simulink model "satcorr_108"  (Simulink 6.2)
settings: Solver=ode45  StartTime=0.0  StopTime=5000  RelTol=1e-3
undefined symbols (not defined in the file): cmult_4bit_br, cmult_4bit_em, cmult_4bit_sl
libraries: xbsIndex_r3 x473, casper_library x42, xps_library x31, ddc_library x4, fft_library x2, pfb_library x2, simulink x1
(part 1 of 5)
settings Model: LastModifiedBy=siemion
settings DebuggingCC: SolverPrmCheckMsg=warning

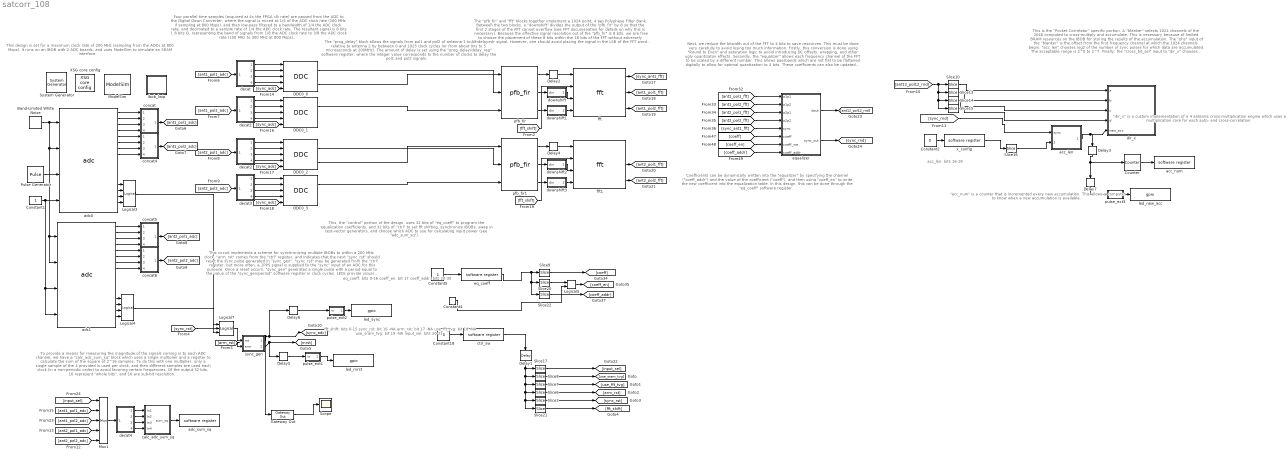
== system satcorr_108 ==
  note: fft_shift: bits 0-15
      | sync_rst: bit 16 -NA
      | arm_rst: bit 17 -NA
      | use_fft_tvg: bit 18 -NA
      | use_sram_tvg: bit 19 -NA
      | input_sel: bits 20-21
  note: acc_len: bits 16-18
  note: eq_coeff: bits 0-16
      | coeff_en: bit 17
      | coeff_addr: bits 20-30
  note: This design is set for a maximum
      | clock rate of 200 MHz (sampling
      | from the ADCs at 800 Mxps).  It
      | runs on an IBOB with 2 ADC boards,
      | and uses ModelSim to simulate an
      | SRAM interface.
  note: This circuit implements a scheme for synchronizing
      | multiple IBOBs to within a 200 MHz clock.  "arm_rst"
      | comes from the "ctrl" register, and indicates that the
      | next "sync_rst" should reset the sync pulse generated
      | in "sync_gen".  "sync_rst" may be generated from
      | the "ctrl" register, but more often, a 1PPS signal is
      | supplied to the "sync" input of an ADC for this
      | purpose.  Once a reset occurs, "sync_gen" generates
      | a single pulse with a period equal to the value
      | of the "sync_gen/period" software register in clock
      | cycles. LEDs provide visual confirmation that an arm and
      | reset occur.
  note: Four parallel time samples (acquired at 4x the
      | FPGA clk rate) are passed from the ADC to the
      | Digital Down Converter, where the signal is mixed
      | at 1/4 of the ADC clock rate (200 MHz if sampling
      | at 800 Msps), and then low-pass filtered to a
      | bandwidth of 1/4 the ADC clock rate, and decimated
      | to a sample rate of 1/4 the ADC clock rate.  The
      | resultant signal is 8 bits I, 8 bits Q, representing the
      | band of signals from 1/8 the ADC clock rate to
      | 3/8 the ADC clock rate (100 MHz to 300 MHz at
      | 800 Msps).
  note: The "pfb_fir" and "fft" blocks together implement a 1024 point,
      | 4 tap Polyphase Filter Bank.  Between the two blocks, a "downshift"
      | divides the output of the "pfb_fir" by 8 so that the first 2 stages of
      | the FFT cannot overflow (see FFT documenation for details on why
      | this is necessary).  Because the effective signal resolution out of
      | the "pfb_fir" is 8 bits, we are free to choose the placement of
      | these 8 bits within the 18 bits of the FFT without adversely affecting
      | our signal.  However, one should avoid placing the signal in the LSB
      | of the FFT word because of rounding effects.  Thus, we downshift
      | only 3 bits.
  note: Next, we reduce the bitwidth out of the FFT to 4 bits to save resources.
      | This must be done very carefully to avoid losing too much information.
      | Firstly, this conversion is done using "Round to Even" and saturation
      | logic to avoid introducing DC offsets, wrapping, and other ugly quantizaton
      | effects.  Secondly, the "equalizer" allows each frequency channel of the
      | FFT to be scaled by a different number.  This allows passbands which are
      | not flat to be flattened digitally to allow for optimal quantization to 4 bits.
      | These coefficients can also be updated dynamically for gain control.
  note: Coefficients can be dynamically written into the "equalizer" by
      | specifying the channel ("coeff_addr") and the value of the
      | coefficient ("coeff"), and then using "coeff_en" to write the
      | new coefficient into the equalization table.  In this design,
      | this can be done through the "eq_coeff" software
      | register.
  note: To provide a means for measuring the magnitude of the signals
      | coming in to each ADC channel, we have a "calc_adc_sum_sq"
      | block which uses a single multiplier and a regsiter to calculate
      | the sum of the square of 2^16 samples.  To do this with one
      | multiplier, only a single sample of the 4 provided is used
      | per clock, and then different samples are used each clock (in
      | a non-periodic order) to avoid favoring certain frequencies.
      | Of the output 32 bits, 16 represent "whole bits", and 16
      | are sub-bit resolution.
  note: This is the "Pocket Correlator" specific portion.  A "blanker" selects
      | 1024 channels of the 2048 computed to cross-multiply and accumulate.
      | This is necessary because of limited BRAM resources on the IBOB
      | for storing the results of the accumulation.  The "phs" input of the "blanker"
      | is the offset from the first frequency channel at which the 1024 channels begin.
      | "acc_len" chooses log2 of the  number of sync pulses for which data are
      | accumulated.  The acceptable range is 2^0 to 2^7.  Finally, the "cross_bit_sel"
      | input to "dir_x" chooses which 16 bits of the 32 accumulated bits are written
      | to the BRAM output buffer.  Only 16 bits real, 16 imag are passed along
      | to reduce download time over the serial cable to a computer.  Which 16 of
      | the 32 computed bits are passed along needs to be selectable because
      | highly correlated signals will accumulate to much larger values than
      | uncorrelated signals.  Values of "cross_bit_sel" can be 0,1,2 or 3
      | corresponding to offsets of 4, 8, 12, and 16 bits from the LSB.
  note: "dir_x" is a custom implementation
      | of a 4 antenna cross-multiplication
      | engine which uses a multiplication
      | core for each auto- and cross-correlation.
  note: "acc_num" is a counter that is
      | incremented every new accumulation.
      | This allows a computer to know when
      | a new accumulation is available.
  note: This, the "control" portion of the design, uses
      | 32 bits of "eq_coeff" to program the equalization
      | coefficients, and 32 bits of "ctrl" to set fft shifting,
      | synchronize IBOBs, swap in test-vector generators,
      | and choose which ADC to use for calculating
      | input power (see "adc_sum_sq").
  note: The "prog_delay" block allows the signals from pol1 and pol2 of antenna 1 to be
      | delayed relative to antenna 2 by between 0 and 1023 clock cycles (or from about
      | 0ns to 5 microseconds at 200MHz).  The amount of delay is set using the
      | "prog_delay/delay_reg" software register, where the integer value corresponds to
      | the number of clocks to delay the pol1 and pol2 signals.
  " System Generator" : xbsIndex_r3/ System Generator  Tag=genX  xilinxfamily=Virtex2P  part=xc2vp50  speed=-7  package=ff1152  synthesis_tool=XST  directory=./satcorr_1/sysgen  testbench=off  simulink_period=1  sysclk_period=41.6667  incr_netlist=off  trim_vbits=Everywhere in SubSystem  dbl_ovrd=According to Block Masks  core_generation=According to Block Masks  run_coregen=off  deprecated_control=off  eval_field=0
      settings: AttributesFormatString=System\nGenerator
  Band-Limited White Noise : simulink/Sources/Band-Limited White Noise  Cov=[0.1]  Ts=0.1  seed=[23341]
  Constant1 : Constant
  Constant18 : Constant  Value=0
  Constant2 : Constant  Value=0
  Constant4 : xbsIndex_r3/Constant  const=1  equ=P=C  arith_type=Boolean  n_bits=1  bin_pt=0  opselect=C  inp2=PCIN>>17  opr=+  inp1=P  carry=CIN  iostate=0  explicit_period=on  period=1  dbl_ovrd=off
  Constant5 : Constant
  Counter : xbsIndex_r3/Counter  cnt_type=Free Running  n_bits=32  bin_pt=0  arith_type=Unsigned  start_count=0  cnt_to=Inf  cnt_by_val=1  operation=Up  explicit_period=off  period=1  load_pin=off  rst=off  en=on  dbl_ovrd=off  show_param=off  use_rpm=on  gen_core=off
      settings: xl_area=[0, 0, 0, 0, 0, 0, 0]
  DDC0_{0..3} (4 alike) : ddc_library/DDC  freq_div=4  lo_freq=1  num_inputs=4  lo_bitwidth=8  lpfir_coeff=".9 * [-0.0161   -0.0428   -0.0504   -0.0249    0.0354    0.1170    0.1948    0.2422    0.2422    0.1948    0.1170  0.0354   -0.0249   -0.0504   -0.0428   -0.0161]"  BitWidthOut=8  quantization="Round  (unbiased: Even Values)"  add_latency=2  mult_latency=4
  Delay1 : xbsIndex_r3/Delay  Orientation=down  latency=1  reg_retiming=off  explicit_period=off  period=1  en=off  accept_only_valid=off  init_zero=on  dbl_ovrd=off  show_param=off
      settings: xl_area=[0, 0, 0, 0, 0, 0, 0]
  Delay2 : xbsIndex_r3/Delay  latency=2  reg_retiming=off  explicit_period=off  period=1  en=off  accept_only_valid=off  init_zero=on  dbl_ovrd=off  show_param=off
      settings: xl_area=[0, 0, 0, 0, 0, 0, 0]
  Delay3 : xbsIndex_r3/Delay  Orientation=down  latency=4  reg_retiming=on  explicit_period=off  period=1  en=off  accept_only_valid=off  init_zero=on  dbl_ovrd=off  show_param=on
      settings: xl_area=[0, 0, 0, 0, 0, 0, 0]
  Delay4 : xbsIndex_r3/Delay  latency=2  reg_retiming=off  explicit_period=off  period=1  en=off  accept_only_valid=off  init_zero=on  dbl_ovrd=off  show_param=off
      settings: xl_area=[0, 0, 0, 0, 0, 0, 0]
  Delay5 : xbsIndex_r3/Delay  latency=2  reg_retiming=on  explicit_period=off  period=1  en=off  accept_only_valid=off  init_zero=on  dbl_ovrd=off  show_param=off
      settings: xl_area=[0, 0, 0, 0, 0, 0, 0]
  Delay6 : xbsIndex_r3/Delay  latency=2  reg_retiming=on  explicit_period=off  period=1  en=off  accept_only_valid=off  init_zero=on  dbl_ovrd=off  show_param=off
      settings: xl_area=[0, 0, 0, 0, 0, 0, 0]
  Delay7 : xbsIndex_r3/Delay  Orientation=down  latency=2  reg_retiming=on  explicit_period=off  period=1  en=off  accept_only_valid=off  init_zero=on  dbl_ovrd=off  show_param=off
      settings: xl_area=[0, 0, 0, 0, 0, 0, 0]
  Gateway Out : xbsIndex_r3/Gateway Out  output_type=Double  nbits=8  bin_pt=6  arith_type=Boolean  quantization=Truncate  overflow=Wrap  hdl_port=on  timing_constraint=None  locs_specified=off  LOCs={}  needs_fixed_name=off  show_param=off
      settings: xl_area=[0, 0, 0, 0, 0, 0, 0]
  Logical3 : xbsIndex_r3/Logical  logical_function=OR  inputs=4  precision=Full  arith_type=Unsigned  n_bits=8  bin_pt=2  align_bp=on  latency=2  explicit_period=off  period=1  en=off  dbl_ovrd=off  show_param=off
      settings: xl_area=[0, 0, 0, 0, 0, 0, 0]
  Logical4 : xbsIndex_r3/Logical  logical_function=OR  inputs=4  precision=Full  arith_type=Unsigned  n_bits=8  bin_pt=2  align_bp=on  latency=2  explicit_period=off  period=1  en=off  dbl_ovrd=off  show_param=off
      settings: xl_area=[0, 0, 0, 0, 0, 0, 0]
  Logical5 : xbsIndex_r3/Logical  logical_function=AND  inputs=2  precision=Full  arith_type=Unsigned  n_bits=8  bin_pt=2  align_bp=on  latency=0  explicit_period=off  period=1  en=off  dbl_ovrd=off  show_param=off
      settings: xl_area=[0, 0, 0, 0, 0, 0, 0]
  Logical7 : xbsIndex_r3/Logical  logical_function=OR  inputs=3  precision=Full  arith_type=Unsigned  n_bits=8  bin_pt=2  align_bp=on  latency=1  explicit_period=off  period=1  en=off  dbl_ovrd=off  show_param=off
      settings: xl_area=[0, 0, 0, 0, 0, 0, 0]
  ModelSim : xbsIndex_r3/ModelSim  dir=./modelsim  waveform=on  leave_open=on  skip_compile=off  custom_scripts=off  startup_timeout=40
  Mux1 : xbsIndex_r3/Mux  inputs=4  precision=Full  arith_type="Signed  (2's comp)"  n_bits=8  bin_pt=2  quantization=Truncate  overflow=Wrap  latency=2  explicit_period=on  period=1  en=off  dbl_ovrd=off  show_param=off  mux_type=off  use_rpm=off  gen_core=off
      settings: xl_area=[0, 0, 0, 0, 0, 0, 0]
  Pulse Generator : DiscretePulseGenerator  Period=2^27
  Scope : Scope
      settings: YMin=-1  YMax=1
  Slice10 : xbsIndex_r3/Slice  mode=Lower Bit Location + Width  nbits=8  bit1=0  base1=MSB of Input  bit0=24  base0=LSB of Input  boolean_output=off  explicit_period=off  period=1  dbl_ovrd=off
  Slice13 : xbsIndex_r3/Slice  mode=Lower Bit Location + Width  nbits=8  bit1=0  base1=MSB of Input  bit0=16  base0=LSB of Input  boolean_output=off  explicit_period=off  period=1  dbl_ovrd=off
  Slice14 : xbsIndex_r3/Slice  mode=Lower Bit Location + Width  nbits=8  bit1=0  base1=MSB of Input  bit0=8  base0=LSB of Input  boolean_output=off  explicit_period=off  period=1  dbl_ovrd=off
  Slice15 : xbsIndex_r3/Slice  mode=Lower Bit Location + Width  nbits=8  bit1=0  base1=MSB of Input  bit0=0  base0=LSB of Input  boolean_output=off  explicit_period=off  period=1  dbl_ovrd=off
  Slice16 : xbsIndex_r3/Slice  mode=Lower Bit Location + Width  nbits=3  bit1=0  base1=MSB of Input  bit0=16  base0=LSB of Input  boolean_output=off  explicit_period=off  period=1  dbl_ovrd=off
  Slice17 : xbsIndex_r3/Slice  mode=Lower Bit Location + Width  nbits=2  bit1=0  base1=MSB of Input  bit0=20  base0=LSB of Input  boolean_output=off  explicit_period=off  period=1  dbl_ovrd=off
  Slice20 : xbsIndex_r3/Slice  mode=Lower Bit Location + Width  nbits=1  bit1=0  base1=MSB of Input  bit0=17  base0=LSB of Input  boolean_output=on  explicit_period=off  period=1  dbl_ovrd=off
  Slice21 : xbsIndex_r3/Slice  mode=Lower Bit Location + Width  nbits=16  bit1=0  base1=MSB of Input  bit0=0  base0=LSB of Input  boolean_output=off  explicit_period=off  period=1  dbl_ovrd=off
  Slice22 : xbsIndex_r3/Slice  mode=Lower Bit Location + Width  nbits=10  bit1=0  base1=MSB of Input  bit0=20  base0=LSB of Input  boolean_output=off  explicit_period=off  period=1  dbl_ovrd=off
  Slice3 : xbsIndex_r3/Slice  mode=Lower Bit Location + Width  nbits=1  bit1=0  base1=MSB of Input  bit0=16  base0=LSB of Input  boolean_output=on  explicit_period=off  period=1  dbl_ovrd=off
  Slice6 : xbsIndex_r3/Slice  mode=Lower Bit Location + Width  nbits=1  bit1=0  base1=MSB of Input  bit0=17  base0=LSB of Input  boolean_output=on  explicit_period=off  period=1  dbl_ovrd=off
  Slice7 : xbsIndex_r3/Slice  mode=Lower Bit Location + Width  nbits=1  bit1=0  base1=MSB of Input  bit0=18  base0=LSB of Input  boolean_output=off  explicit_period=off  period=1  dbl_ovrd=off
  Slice8 : xbsIndex_r3/Slice  mode=Lower Bit Location + Width  nbits=1  bit1=0  base1=MSB of Input  bit0=19  base0=LSB of Input  boolean_output=off  explicit_period=off  period=1  dbl_ovrd=off
  Slice9 : xbsIndex_r3/Slice  mode=Lower Bit Location + Width  nbits=17  bit1=0  base1=MSB of Input  bit0=0  base0=LSB of Input  boolean_output=off  explicit_period=off  period=1  dbl_ovrd=off
  XSG core config : xps_library/XSG core config  Tag=xps:xsg  hw_sys=iBOB  ibob_linux=off  clk_src=adc0_clk  gpio_clk_io_group=iBOB:sma  gpio_clk_bit_index=0  clk_rate=27  sample_period=1  synthesis_tool=XST  mpc_type=powerpc405
  acc_len : Subsystem
  acc_num : xps_library/software register  Tag=xps:sw_reg  io_dir=To Processor  arith_type=Unsigned  bitwidth=32  bin_pt=0  sample_period=1  gw_name=satcorr_1_acc_num_user_data_in
  adc0 : xps_library/adc  Tag=xps:adc  adc_brd=iBOB:adc0  adc_clk_rate=108  adc_interleave=off  sample_period=1
  adc1 : xps_library/adc  Tag=xps:adc  adc_brd=iBOB:adc1  adc_clk_rate=108  adc_interleave=off  sample_period=1
  adc_sum_sq : xps_library/software register  Tag=xps:sw_reg  io_dir=To Processor  arith_type=Unsigned  bitwidth=32  bin_pt=14  sample_period=1  gw_name=satcorr_1_adc_sum_sq_user_data_in
  calc_adc_sum_sq : Subsystem
  concat : Subsystem
  concat4 : Subsystem
  concat5 : Subsystem
  concat6 : Subsystem
  ctrl_sw : xps_library/software register  Tag=xps:sw_reg  io_dir=From Processor  arith_type=Unsigned  bitwidth=32  bin_pt=0  sample_period=1  gw_name=satcorr_1_ctrl_sw_user_data_out
  decat : Subsystem
  decat1 : Subsystem
  decat2 : Subsystem
  decat3 : Subsystem
  decat4 : Subsystem
  dir_x : Subsystem
  downshift : Subsystem
  downshift1 : Subsystem
  downshift2 : Subsystem
  downshift3 : Subsystem
  eq_coeff : xps_library/software register  Tag=xps:sw_reg  io_dir=From Processor  arith_type=Unsigned  bitwidth=32  bin_pt=0  sample_period=1  gw_name=satcorr_1_eq_coeff_user_data_out
  equalizer : Subsystem
  fft : fft_library/fft  FFTSize=10  BitWidth=18  n_inputs=0  quantization="Round  (unbiased: Even Values)"  overflow=Wrap  add_latency=1  mult_latency=2  bram_latency=2
  fft1 : fft_library/fft  FFTSize=10  BitWidth=18  n_inputs=0  quantization="Round  (unbiased: Even Values)"  overflow=Wrap  add_latency=1  mult_latency=2  bram_latency=2
  ibob_lwip : Subsystem  AncestorBlock=xps_library/ibob_lwip
      mask Type: ibobethlite
      mask Description: Attaches SRAM0 to the PLB bus and adds LWIP support.
      mask Display: fprintf('IBOB\nLWIP');
  led_mrst : xps_library/gpio  Tag=xps:gpio  io_group=iBOB:led  io_dir=out  arith_type=Boolean  bitwidth=1  bin_pt=0  bit_index=3  sample_period=1  use_ddr=off  reg_iob=off  reg_clk_phase=0  termination=None
  led_new_acc : xps_library/gpio  Tag=xps:gpio  io_group=iBOB:led  io_dir=out  arith_type=Boolean  bitwidth=1  bin_pt=0  bit_index=5  sample_period=1  use_ddr=off  reg_iob=off  reg_clk_phase=0  termination=None
  led_sync : xps_library/gpio  Tag=xps:gpio  io_group=iBOB:led  io_dir=out  arith_type=Boolean  bitwidth=1  bin_pt=0  bit_index=2  sample_period=1  use_ddr=off  reg_iob=off  reg_clk_phase=0  termination=None
  pfb_fir : pfb_library/pfb_fir  PFBSize=10  TotalTaps=4  WindowType=hamming  n_inputs=0  MakeBiplex=on  BitWidthIn=8  BitWidthOut=18  CoeffBitWidth=8  CoeffDistMem=off  add_latency=1  mult_latency=2  bram_latency=2  quantization="Round  (unbiased: Even Values)"  fwidth=1
      link override pol1_in1_first_tap/sync_delay/Constant: equ=P=C
      link override pol1_in1_first_tap/sync_delay/Constant1: equ=P=C
      link override pol1_in1_first_tap/sync_delay/Constant2: equ=P=C
      link override pol1_in1_first_tap/sync_delay/Constant3: equ=P=C
      link override pol1_in1_tap10/sync_delay/Constant: equ=P=C
      link override pol1_in1_tap10/sync_delay/Constant1: equ=P=C
      link override pol1_in1_tap10/sync_delay/Constant2: equ=P=C
      link override pol1_in1_tap10/sync_delay/Constant3: equ=P=C
      link override pol1_in1_tap11/sync_delay/Constant: equ=P=C
      link override pol1_in1_tap11/sync_delay/Constant1: equ=P=C
      link override pol1_in1_tap11/sync_delay/Constant2: equ=P=C
      link override pol1_in1_tap11/sync_delay/Constant3: equ=P=C
      link override pol1_in1_tap12/sync_delay/Constant: equ=P=C
      link override pol1_in1_tap12/sync_delay/Constant1: equ=P=C
      link override pol1_in1_tap12/sync_delay/Constant2: equ=P=C
      link override pol1_in1_tap12/sync_delay/Constant3: equ=P=C
      link override pol1_in1_tap13/sync_delay/Constant: equ=P=C
      link override pol1_in1_tap13/sync_delay/Constant1: equ=P=C
      link override pol1_in1_tap13/sync_delay/Constant2: equ=P=C
      link override pol1_in1_tap13/sync_delay/Constant3: equ=P=C
      link override pol1_in1_tap14/sync_delay/Constant: equ=P=C
      link override pol1_in1_tap14/sync_delay/Constant1: equ=P=C
      link override pol1_in1_tap14/sync_delay/Constant2: equ=P=C
      link override pol1_in1_tap14/sync_delay/Constant3: equ=P=C
      link override pol1_in1_tap15/sync_delay/Constant: equ=P=C
      link override pol1_in1_tap15/sync_delay/Constant1: equ=P=C
      link override pol1_in1_tap15/sync_delay/Constant2: equ=P=C
      link override pol1_in1_tap15/sync_delay/Constant3: equ=P=C
      link override pol1_in1_tap2/sync_delay/Constant: equ=P=C
      link override pol1_in1_tap2/sync_delay/Constant1: equ=P=C
      link override pol1_in1_tap2/sync_delay/Constant2: equ=P=C
      link override pol1_in1_tap2/sync_delay/Constant3: equ=P=C
      link override pol1_in1_tap3/sync_delay/Constant: equ=P=C
      link override pol1_in1_tap3/sync_delay/Constant1: equ=P=C
      link override pol1_in1_tap3/sync_delay/Constant2: equ=P=C
      link override pol1_in1_tap3/sync_delay/Constant3: equ=P=C
      link override pol1_in1_tap4/sync_delay/Constant: equ=P=C
      link override pol1_in1_tap4/sync_delay/Constant1: equ=P=C
      link override pol1_in1_tap4/sync_delay/Constant2: equ=P=C
      link override pol1_in1_tap4/sync_delay/Constant3: equ=P=C
      link override pol1_in1_tap5/sync_delay/Constant: equ=P=C
      link override pol1_in1_tap5/sync_delay/Constant1: equ=P=C
      link override pol1_in1_tap5/sync_delay/Constant2: equ=P=C
      link override pol1_in1_tap5/sync_delay/Constant3: equ=P=C
      link override pol1_in1_tap6/sync_delay/Constant: equ=P=C
      link override pol1_in1_tap6/sync_delay/Constant1: equ=P=C
      link override pol1_in1_tap6/sync_delay/Constant2: equ=P=C
      link override pol1_in1_tap6/sync_delay/Constant3: equ=P=C
      link override pol1_in1_tap7/sync_delay/Constant: equ=P=C
      link override pol1_in1_tap7/sync_delay/Constant1: equ=P=C
      link override pol1_in1_tap7/sync_delay/Constant2: equ=P=C
      link override pol1_in1_tap7/sync_delay/Constant3: equ=P=C
      link override pol1_in1_tap8/sync_delay/Constant: equ=P=C
      link override pol1_in1_tap8/sync_delay/Constant1: equ=P=C
      link override pol1_in1_tap8/sync_delay/Constant2: equ=P=C
      link override pol1_in1_tap8/sync_delay/Constant3: equ=P=C
      link override pol1_in1_tap9/sync_delay/Constant: equ=P=C
      link override pol1_in1_tap9/sync_delay/Constant1: equ=P=C
      link override pol1_in1_tap9/sync_delay/Constant2: equ=P=C
      link override pol1_in1_tap9/sync_delay/Constant3: equ=P=C
      link override pol2_in1_first_tap/sync_delay/Constant: equ=P=C
      link override pol2_in1_first_tap/sync_delay/Constant1: equ=P=C
      link override pol2_in1_first_tap/sync_delay/Constant2: equ=P=C
      link override pol2_in1_first_tap/sync_delay/Constant3: equ=P=C
      link override pol2_in1_tap10/sync_delay/Constant: equ=P=C
      link override pol2_in1_tap10/sync_delay/Constant1: equ=P=C
      link override pol2_in1_tap10/sync_delay/Constant2: equ=P=C
      link override pol2_in1_tap10/sync_delay/Constant3: equ=P=C
      link override pol2_in1_tap11/sync_delay/Constant: equ=P=C
      link override pol2_in1_tap11/sync_delay/Constant1: equ=P=C
      link override pol2_in1_tap11/sync_delay/Constant2: equ=P=C
      link override pol2_in1_tap11/sync_delay/Constant3: equ=P=C
      link override pol2_in1_tap12/sync_delay/Constant: equ=P=C
      link override pol2_in1_tap12/sync_delay/Constant1: equ=P=C
      link override pol2_in1_tap12/sync_delay/Constant2: equ=P=C
      link override pol2_in1_tap12/sync_delay/Constant3: equ=P=C
      link override pol2_in1_tap13/sync_delay/Constant: equ=P=C
      link override pol2_in1_tap13/sync_delay/Constant1: equ=P=C
      link override pol2_in1_tap13/sync_delay/Constant2: equ=P=C
      link override pol2_in1_tap13/sync_delay/Constant3: equ=P=C
      link override pol2_in1_tap14/sync_delay/Constant: equ=P=C
      link override pol2_in1_tap14/sync_delay/Constant1: equ=P=C
      link override pol2_in1_tap14/sync_delay/Constant2: equ=P=C
      link override pol2_in1_tap14/sync_delay/Constant3: equ=P=C
      link override pol2_in1_tap15/sync_delay/Constant: equ=P=C
      link override pol2_in1_tap15/sync_delay/Constant1: equ=P=C
      link override pol2_in1_tap15/sync_delay/Constant2: equ=P=C
      link override pol2_in1_tap15/sync_delay/Constant3: equ=P=C
      link override pol2_in1_tap2/sync_delay/Constant: equ=P=C
      link override pol2_in1_tap2/sync_delay/Constant1: equ=P=C
      link override pol2_in1_tap2/sync_delay/Constant2: equ=P=C
      link override pol2_in1_tap2/sync_delay/Constant3: equ=P=C
      link override pol2_in1_tap3/sync_delay/Constant: equ=P=C
      link override pol2_in1_tap3/sync_delay/Constant1: equ=P=C
      link override pol2_in1_tap3/sync_delay/Constant2: equ=P=C
      link override pol2_in1_tap3/sync_delay/Constant3: equ=P=C
      link override pol2_in1_tap4/sync_delay/Constant: equ=P=C
      link override pol2_in1_tap4/sync_delay/Constant1: equ=P=C
      link override pol2_in1_tap4/sync_delay/Constant2: equ=P=C
      link override pol2_in1_tap4/sync_delay/Constant3: equ=P=C
      link override pol2_in1_tap5/sync_delay/Constant: equ=P=C
      link override pol2_in1_tap5/sync_delay/Constant1: equ=P=C
      link override pol2_in1_tap5/sync_delay/Constant2: equ=P=C
      link override pol2_in1_tap5/sync_delay/Constant3: equ=P=C
      link override pol2_in1_tap6/sync_delay/Constant: equ=P=C
      link override pol2_in1_tap6/sync_delay/Constant1: equ=P=C
      link override pol2_in1_tap6/sync_delay/Constant2: equ=P=C
      link override pol2_in1_tap6/sync_delay/Constant3: equ=P=C
      link override pol2_in1_tap7/sync_delay/Constant: equ=P=C
      link override pol2_in1_tap7/sync_delay/Constant1: equ=P=C
      link override pol2_in1_tap7/sync_delay/Constant2: equ=P=C
      link override pol2_in1_tap7/sync_delay/Constant3: equ=P=C
      link override pol2_in1_tap8/sync_delay/Constant: equ=P=C
      link override pol2_in1_tap8/sync_delay/Constant1: equ=P=C
      link override pol2_in1_tap8/sync_delay/Constant2: equ=P=C
      link override pol2_in1_tap8/sync_delay/Constant3: equ=P=C
      link override pol2_in1_tap9/sync_delay/Constant: equ=P=C
      link override pol2_in1_tap9/sync_delay/Constant1: equ=P=C
      link override pol2_in1_tap9/sync_delay/Constant2: equ=P=C
      link override pol2_in1_tap9/sync_delay/Constant3: equ=P=C
  pfb_fir1 : pfb_library/pfb_fir  PFBSize=10  TotalTaps=4  WindowType=hamming  n_inputs=0  MakeBiplex=on  BitWidthIn=8  BitWidthOut=18  CoeffBitWidth=8  CoeffDistMem=off  add_latency=1  mult_latency=2  bram_latency=2  quantization="Round  (unbiased: Even Values)"  fwidth=1
      link override pol1_in1_first_tap/sync_delay/Constant: equ=P=C
      link override pol1_in1_first_tap/sync_delay/Constant1: equ=P=C
      link override pol1_in1_first_tap/sync_delay/Constant2: equ=P=C
      link override pol1_in1_first_tap/sync_delay/Constant3: equ=P=C
      link override pol1_in1_tap10/sync_delay/Constant: equ=P=C
      link override pol1_in1_tap10/sync_delay/Constant1: equ=P=C
      link override pol1_in1_tap10/sync_delay/Constant2: equ=P=C
      link override pol1_in1_tap10/sync_delay/Constant3: equ=P=C
      link override pol1_in1_tap11/sync_delay/Constant: equ=P=C
      link override pol1_in1_tap11/sync_delay/Constant1: equ=P=C
      link override pol1_in1_tap11/sync_delay/Constant2: equ=P=C
      link override pol1_in1_tap11/sync_delay/Constant3: equ=P=C
      link override pol1_in1_tap12/sync_delay/Constant: equ=P=C
      link override pol1_in1_tap12/sync_delay/Constant1: equ=P=C
      link override pol1_in1_tap12/sync_delay/Constant2: equ=P=C
      link override pol1_in1_tap12/sync_delay/Constant3: equ=P=C
      link override pol1_in1_tap13/sync_delay/Constant: equ=P=C
      link override pol1_in1_tap13/sync_delay/Constant1: equ=P=C
      link override pol1_in1_tap13/sync_delay/Constant2: equ=P=C
      link override pol1_in1_tap13/sync_delay/Constant3: equ=P=C
      link override pol1_in1_tap14/sync_delay/Constant: equ=P=C
      link override pol1_in1_tap14/sync_delay/Constant1: equ=P=C
      link override pol1_in1_tap14/sync_delay/Constant2: equ=P=C
      link override pol1_in1_tap14/sync_delay/Constant3: equ=P=C
      link override pol1_in1_tap15/sync_delay/Constant: equ=P=C
      link override pol1_in1_tap15/sync_delay/Constant1: equ=P=C
      link override pol1_in1_tap15/sync_delay/Constant2: equ=P=C
      link override pol1_in1_tap15/sync_delay/Constant3: equ=P=C
      link override pol1_in1_tap2/sync_delay/Constant: equ=P=C
      link override pol1_in1_tap2/sync_delay/Constant1: equ=P=C
      link override pol1_in1_tap2/sync_delay/Constant2: equ=P=C
      link override pol1_in1_tap2/sync_delay/Constant3: equ=P=C
      link override pol1_in1_tap3/sync_delay/Constant: equ=P=C
      link override pol1_in1_tap3/sync_delay/Constant1: equ=P=C
      link override pol1_in1_tap3/sync_delay/Constant2: equ=P=C
      link override pol1_in1_tap3/sync_delay/Constant3: equ=P=C
      link override pol1_in1_tap4/sync_delay/Constant: equ=P=C
      link override pol1_in1_tap4/sync_delay/Constant1: equ=P=C
      link override pol1_in1_tap4/sync_delay/Constant2: equ=P=C
      link override pol1_in1_tap4/sync_delay/Constant3: equ=P=C
      link override pol1_in1_tap5/sync_delay/Constant: equ=P=C
      link override pol1_in1_tap5/sync_delay/Constant1: equ=P=C
      link override pol1_in1_tap5/sync_delay/Constant2: equ=P=C
      link override pol1_in1_tap5/sync_delay/Constant3: equ=P=C
      link override pol1_in1_tap6/sync_delay/Constant: equ=P=C
      link override pol1_in1_tap6/sync_delay/Constant1: equ=P=C
      link override pol1_in1_tap6/sync_delay/Constant2: equ=P=C
      link override pol1_in1_tap6/sync_delay/Constant3: equ=P=C
      link override pol1_in1_tap7/sync_delay/Constant: equ=P=C
      link override pol1_in1_tap7/sync_delay/Constant1: equ=P=C
      link override pol1_in1_tap7/sync_delay/Constant2: equ=P=C
      link override pol1_in1_tap7/sync_delay/Constant3: equ=P=C
      link override pol1_in1_tap8/sync_delay/Constant: equ=P=C
      link override pol1_in1_tap8/sync_delay/Constant1: equ=P=C
      link override pol1_in1_tap8/sync_delay/Constant2: equ=P=C
      link override pol1_in1_tap8/sync_delay/Constant3: equ=P=C
      link override pol1_in1_tap9/sync_delay/Constant: equ=P=C
      link override pol1_in1_tap9/sync_delay/Constant1: equ=P=C
      link override pol1_in1_tap9/sync_delay/Constant2: equ=P=C
      link override pol1_in1_tap9/sync_delay/Constant3: equ=P=C
      link override pol2_in1_first_tap/sync_delay/Constant: equ=P=C
      link override pol2_in1_first_tap/sync_delay/Constant1: equ=P=C
      link override pol2_in1_first_tap/sync_delay/Constant2: equ=P=C
      link override pol2_in1_first_tap/sync_delay/Constant3: equ=P=C
      link override pol2_in1_tap10/sync_delay/Constant: equ=P=C
      link override pol2_in1_tap10/sync_delay/Constant1: equ=P=C
      link override pol2_in1_tap10/sync_delay/Constant2: equ=P=C
      link override pol2_in1_tap10/sync_delay/Constant3: equ=P=C
      link override pol2_in1_tap11/sync_delay/Constant: equ=P=C
      link override pol2_in1_tap11/sync_delay/Constant1: equ=P=C
      link override pol2_in1_tap11/sync_delay/Constant2: equ=P=C
      link override pol2_in1_tap11/sync_delay/Constant3: equ=P=C
      link override pol2_in1_tap12/sync_delay/Constant: equ=P=C
      link override pol2_in1_tap12/sync_delay/Constant1: equ=P=C
      link override pol2_in1_tap12/sync_delay/Constant2: equ=P=C
      link override pol2_in1_tap12/sync_delay/Constant3: equ=P=C
      link override pol2_in1_tap13/sync_delay/Constant: equ=P=C
      link override pol2_in1_tap13/sync_delay/Constant1: equ=P=C
      link override pol2_in1_tap13/sync_delay/Constant2: equ=P=C
      link override pol2_in1_tap13/sync_delay/Constant3: equ=P=C
      link override pol2_in1_tap14/sync_delay/Constant: equ=P=C
      link override pol2_in1_tap14/sync_delay/Constant1: equ=P=C
      link override pol2_in1_tap14/sync_delay/Constant2: equ=P=C
      link override pol2_in1_tap14/sync_delay/Constant3: equ=P=C
      link override pol2_in1_tap15/sync_delay/Constant: equ=P=C
      link override pol2_in1_tap15/sync_delay/Constant1: equ=P=C
      link override pol2_in1_tap15/sync_delay/Constant2: equ=P=C
      link override pol2_in1_tap15/sync_delay/Constant3: equ=P=C
      link override pol2_in1_tap2/sync_delay/Constant: equ=P=C
      link override pol2_in1_tap2/sync_delay/Constant1: equ=P=C
      link override pol2_in1_tap2/sync_delay/Constant2: equ=P=C
      link override pol2_in1_tap2/sync_delay/Constant3: equ=P=C
      link override pol2_in1_tap3/sync_delay/Constant: equ=P=C
      link override pol2_in1_tap3/sync_delay/Constant1: equ=P=C
      link override pol2_in1_tap3/sync_delay/Constant2: equ=P=C
      link override pol2_in1_tap3/sync_delay/Constant3: equ=P=C
      link override pol2_in1_tap4/sync_delay/Constant: equ=P=C
      link override pol2_in1_tap4/sync_delay/Constant1: equ=P=C
      link override pol2_in1_tap4/sync_delay/Constant2: equ=P=C
      link override pol2_in1_tap4/sync_delay/Constant3: equ=P=C
      link override pol2_in1_tap5/sync_delay/Constant: equ=P=C
      link override pol2_in1_tap5/sync_delay/Constant1: equ=P=C
      link override pol2_in1_tap5/sync_delay/Constant2: equ=P=C
      link override pol2_in1_tap5/sync_delay/Constant3: equ=P=C
      link override pol2_in1_tap6/sync_delay/Constant: equ=P=C
      link override pol2_in1_tap6/sync_delay/Constant1: equ=P=C
      link override pol2_in1_tap6/sync_delay/Constant2: equ=P=C
      link override pol2_in1_tap6/sync_delay/Constant3: equ=P=C
      link override pol2_in1_tap7/sync_delay/Constant: equ=P=C
      link override pol2_in1_tap7/sync_delay/Constant1: equ=P=C
      link override pol2_in1_tap7/sync_delay/Constant2: equ=P=C
      link override pol2_in1_tap7/sync_delay/Constant3: equ=P=C
      link override pol2_in1_tap8/sync_delay/Constant: equ=P=C
      link override pol2_in1_tap8/sync_delay/Constant1: equ=P=C
      link override pol2_in1_tap8/sync_delay/Constant2: equ=P=C
      link override pol2_in1_tap8/sync_delay/Constant3: equ=P=C
      link override pol2_in1_tap9/sync_delay/Constant: equ=P=C
      link override pol2_in1_tap9/sync_delay/Constant1: equ=P=C
      link override pol2_in1_tap9/sync_delay/Constant2: equ=P=C
      link override pol2_in1_tap9/sync_delay/Constant3: equ=P=C
  pulse_ext1 : Subsystem  mask{pulse_len=2^23}
      mask prompts: pulse_len "Length of Pulse"
      mask init:
      | bits = ceil(log2(pulse_len+1));
  pulse_ext2 : Subsystem  mask{pulse_len=2^23}
      mask prompts: pulse_len "Length of Pulse"
      mask init:
      | bits = ceil(log2(pulse_len+1));
  pulse_ext3 : Subsystem  mask{pulse_len=2^23}
      mask prompts: pulse_len "Length of Pulse"
      mask init:
      | bits = ceil(log2(pulse_len+1));
  sync_gen : Subsystem
  x_config : xps_library/software register  Tag=xps:sw_reg  io_dir=From Processor  arith_type=Unsigned  bitwidth=32  bin_pt=0  sample_period=1  gw_name=satcorr_1_x_config_user_data_out
  wires:
  Pulse Generator/1 -> adc0/3
  Constant1/1 -> adc0/4, adc1/4, adc1/3
  Band-Limited White Noise/1 -> adc0/1, adc0/2, adc1/1, adc1/2
  pfb_fir/1 -> Delay2/1
  pfb_fir1/1 -> Delay4/1
  pulse_ext2/1(out) -> led_sync/1
  sync_gen/1(sync) -> [sync_adc], Delay6/1, Gateway Out/1
  pulse_ext1/1(out) -> led_mrst/1
  adc0/13 -> Logical3/1
  adc0/14 -> Logical3/2
  adc0/15 -> Logical3/3
  adc0/16 -> Logical3/4
  adc1/13 -> Logical4/1
  adc1/14 -> Logical4/2
  adc1/15 -> Logical4/3
  adc1/16 -> Logical4/4
  Logical3/1 -> Logical7/1
  Logical7/1 -> sync_gen/1(rst)
  sync_gen/2(mrst) -> [mrst], Delay5/1
  Constant18/1 -> ctrl_sw/1
  ctrl_sw/1 -> Delay1/1
  Slice8/1 -> [use_sram_tvg]
  Slice7/1 -> [use_fft_tvg]
  Slice6/1 -> [arm_rst]
  Slice3/1 -> [sync_rst]
  Slice21/1 -> [fft_shift]
  [arm_rst] -> sync_gen/2(arm)
  decat/1(Out1) -> DDC0_0/1
  decat/2(Out2) -> DDC0_0/2
  decat/3(Out3) -> DDC0_0/3
  decat/4(Out4) -> DDC0_0/4
  adc0/1 -> concat/1(In1)
  adc0/2 -> concat/2(In2)
  adc0/3 -> concat/3(In3)
  adc0/4 -> concat/4(In4)
  concat/1(Out1) -> [ant1_pol1_adc]
  [ant1_pol1_adc] -> decat/1(In1)
  concat4/1(Out1) -> [ant1_pol2_adc]
  adc0/5 -> concat4/1(In1)
  adc0/6 -> concat4/2(In2)
  adc0/7 -> concat4/3(In3)
  adc0/8 -> concat4/4(In4)
  concat5/1(Out1) -> [ant2_pol1_adc]
  concat6/1(Out1) -> [ant2_pol2_adc]
  adc1/1 -> concat5/1(In1)
  adc1/2 -> concat5/2(In2)
  adc1/3 -> concat5/3(In3)
  adc1/4 -> concat5/4(In4)
  adc1/5 -> concat6/1(In1)
  adc1/6 -> concat6/2(In2)
  adc1/7 -> concat6/3(In3)
  adc1/8 -> concat6/4(In4)
  [sync_rst] -> Logical7/2
  Logical4/1 -> Logical7/3
  [ant1_pol2_adc] -> decat1/1(In1)
  decat1/1(Out1) -> DDC0_1/1
  decat1/2(Out2) -> DDC0_1/2
  decat1/3(Out3) -> DDC0_1/3
  decat1/4(Out4) -> DDC0_1/4
  [ant2_pol1_adc] -> decat2/1(In1)
  [ant2_pol2_adc] -> decat3/1(In1)
  decat2/1(Out1) -> DDC0_2/1
  decat2/2(Out2) -> DDC0_2/2
  decat2/3(Out3) -> DDC0_2/3
  decat2/4(Out4) -> DDC0_2/4
  decat3/1(Out1) -> DDC0_3/1
  decat3/2(Out2) -> DDC0_3/2
  decat3/3(Out3) -> DDC0_3/3
  decat3/4(Out4) -> DDC0_3/4
  [sync_adc] -> DDC0_0/5
  [sync_adc] -> DDC0_1/5
  [sync_adc] -> DDC0_2/5
  [sync_adc] -> DDC0_3/5
  [fft_shift] -> fft/2
  [fft_shift] -> fft1/2
  fft/1 -> [sync_ant1_fft]
  fft/2 -> [ant1_pol1_fft]
  fft/3 -> [ant1_pol2_fft]
  fft1/2 -> [ant2_pol1_fft]
  fft1/3 -> [ant2_pol2_fft]
  Constant2/1 -> x_config/1
  x_config/1 -> Slice16/1
  [sync_rnd] -> acc_len/1(sync)
  [ant12_pol12_rnd] -> Slice10/1, Slice15/1, Slice14/1, Slice13/1
  Slice10/1 -> dir_x/1(a)
  Slice13/1 -> dir_x/2(b)
  Slice14/1 -> dir_x/3(c)
  Slice15/1 -> dir_x/4(d)
  acc_len/1(new_acc) -> dir_x/5(new_acc), Delay3/1
  Slice16/1 -> acc_len/2(acc_len)
  pulse_ext3/1(out) -> led_new_acc/1
  Counter/1 -> acc_num/1
  Mux1/1 -> decat4/1(In1)
  decat4/1(Out1) -> calc_adc_sum_sq/1(In1)
  decat4/2(Out2) -> calc_adc_sum_sq/2(In2)
  decat4/3(Out3) -> calc_adc_sum_sq/3(In3)
  decat4/4(Out4) -> calc_adc_sum_sq/4(In4)
  calc_adc_sum_sq/1(sum_sq) -> adc_sum_sq/1
  Slice17/1 -> [input_sel]
  [input_sel] -> Mux1/1
  [ant1_pol1_adc] -> Mux1/2
  [ant1_pol2_adc] -> Mux1/3
  [ant2_pol1_adc] -> Mux1/4
  [ant2_pol2_adc] -> Mux1/5
  Delay1/1 -> Slice8/1, Slice7/1, Slice6/1, Slice3/1, Slice21/1, Slice17/1
  pfb_fir/2 -> downshift/1(din)
  downshift/1(dout) -> fft/3
  pfb_fir/3 -> downshift1/1(din)
  downshift1/1(dout) -> fft/4
  pfb_fir1/2 -> downshift2/1(din)
  downshift2/1(dout) -> fft1/3
  pfb_fir1/3 -> downshift3/1(din)
  downshift3/1(dout) -> fft1/4
  equalizer/1(dout) -> [ant12_pol12_rnd]
  equalizer/2(sync_out) -> [sync_rnd]
  [ant1_pol1_fft] -> equalizer/1(a1p1)
  [ant1_pol2_fft] -> equalizer/2(a1p2)
  [ant2_pol1_fft] -> equalizer/3(a2p1)
  [ant2_pol2_fft] -> equalizer/4(a2p2)
  [sync_ant1_fft] -> equalizer/5(sync)
  Constant4/1 -> Logical5/2
  Constant5/1 -> eq_coeff/1
  eq_coeff/1 -> Slice9/1, Slice22/1, Slice20/1
  Slice20/1 -> Logical5/1
  Slice9/1 -> [coeff]
  Logical5/1 -> [coeff_en]
  [coeff] -> equalizer/6(coeff)
  [coeff_en] -> equalizer/7(coeff_we)
  [coeff_addr] -> equalizer/8(coeff_addr)
  Slice22/1 -> [coeff_addr]
  Delay2/1 -> fft/1
  Delay4/1 -> fft1/1
  Gateway Out/1 -> Scope/1
  Delay3/1 -> Counter/1, Delay7/1
  Delay5/1 -> pulse_ext1/1(in)
  Delay6/1 -> pulse_ext2/1(in)
  Delay7/1 -> pulse_ext3/1(in)
  DDC0_0/2 -> pfb_fir/1
  DDC0_2/2 -> pfb_fir1/1
  DDC0_0/1 -> pfb_fir/2
  DDC0_1/1 -> pfb_fir/3
  DDC0_2/1 -> pfb_fir1/2
  DDC0_3/1 -> pfb_fir1/3

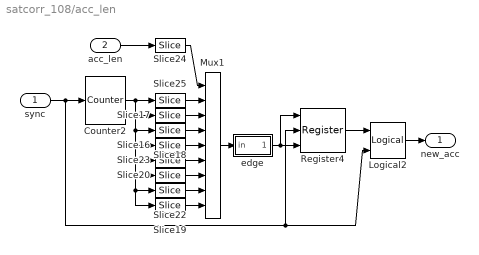
== system satcorr_108/acc_len ==
  sync : Inport  Port=1  LatchInput=off
  acc_len : Inport  Port=2  LatchInput=off
  Counter2 : xbsIndex_r3/Counter  cnt_type=Free Running  n_bits=8  bin_pt=0  arith_type=Unsigned  start_count=0  cnt_to=Inf  cnt_by_val=1  operation=Up  explicit_period=on  period=1  load_pin=off  rst=off  en=on  dbl_ovrd=off  show_param=off  use_rpm=on  gen_core=off
      settings: xl_area=[0, 0, 0, 0, 0, 0, 0]
  Logical2 : xbsIndex_r3/Logical  logical_function=AND  inputs=2  precision=Full  arith_type=Unsigned  n_bits=8  bin_pt=2  align_bp=on  latency=0  explicit_period=off  period=1  en=off  dbl_ovrd=off  show_param=off
      settings: xl_area=[0, 0, 0, 0, 0, 0, 0]
  Mux1 : xbsIndex_r3/Mux  inputs=8  precision=Full  arith_type="Signed  (2's comp)"  n_bits=8  bin_pt=2  quantization=Truncate  overflow=Wrap  latency=1  explicit_period=off  period=1  en=off  dbl_ovrd=off  show_param=off  mux_type=off  use_rpm=off  gen_core=off
      settings: xl_area=[0, 0, 0, 0, 0, 0, 0]
  Register4 : xbsIndex_r3/Register  init=0  reg_only_valid=off  explicit_period=off  period=1  rst=on  en=on  out_en=off  dbl_ovrd=off  show_param=off
      settings: xl_area=[0, 0, 0, 0, 0, 0, 0]
  Slice16 : xbsIndex_r3/Slice  mode=Lower Bit Location + Width  nbits=1  bit1=0  base1=MSB of Input  bit0=3  base0=LSB of Input  boolean_output=on  explicit_period=off  period=1  dbl_ovrd=off
  Slice17 : xbsIndex_r3/Slice  mode=Lower Bit Location + Width  nbits=1  bit1=0  base1=MSB of Input  bit0=1  base0=LSB of Input  boolean_output=on  explicit_period=off  period=1  dbl_ovrd=off
  Slice18 : xbsIndex_r3/Slice  mode=Lower Bit Location + Width  nbits=1  bit1=0  base1=MSB of Input  bit0=2  base0=LSB of Input  boolean_output=on  explicit_period=off  period=1  dbl_ovrd=off
  Slice19 : xbsIndex_r3/Slice  mode=Lower Bit Location + Width  nbits=1  bit1=0  base1=MSB of Input  bit0=7  base0=LSB of Input  boolean_output=on  explicit_period=off  period=1  dbl_ovrd=off
  Slice20 : xbsIndex_r3/Slice  mode=Lower Bit Location + Width  nbits=1  bit1=0  base1=MSB of Input  bit0=5  base0=LSB of Input  boolean_output=on  explicit_period=off  period=1  dbl_ovrd=off
  Slice22 : xbsIndex_r3/Slice  mode=Lower Bit Location + Width  nbits=1  bit1=0  base1=MSB of Input  bit0=6  base0=LSB of Input  boolean_output=on  explicit_period=off  period=1  dbl_ovrd=off
  Slice23 : xbsIndex_r3/Slice  mode=Lower Bit Location + Width  nbits=1  bit1=0  base1=MSB of Input  bit0=4  base0=LSB of Input  boolean_output=on  explicit_period=off  period=1  dbl_ovrd=off
  Slice24 : xbsIndex_r3/Slice  mode=Lower Bit Location + Width  nbits=3  bit1=0  base1=MSB of Input  bit0=0  base0=LSB of Input  boolean_output=off  explicit_period=off  period=1  dbl_ovrd=off
  Slice25 : xbsIndex_r3/Slice  mode=Lower Bit Location + Width  nbits=1  bit1=0  base1=MSB of Input  bit0=0  base0=LSB of Input  boolean_output=on  explicit_period=off  period=1  dbl_ovrd=off
  edge : Subsystem
  new_acc : Outport
  wires:
  Slice22/1 -> Mux1/8
  Slice20/1 -> Mux1/7
  Slice23/1 -> Mux1/6
  Slice16/1 -> Mux1/5
  Slice18/1 -> Mux1/4
  Slice17/1 -> Mux1/3
  Slice25/1 -> Mux1/2
  sync/1 -> Counter2/1, Register4/2, Logical2/2
  acc_len/1 -> Slice24/1
  Counter2/1 -> Slice20/1, Slice22/1, Slice19/1, Slice23/1, Slice16/1, Slice18/1, Slice17/1, Slice25/1
  Slice24/1 -> Mux1/1
  Mux1/1 -> edge/1(in)
  Slice19/1 -> Mux1/9
  edge/1(out) -> Register4/3, Register4/1
  Register4/1 -> Logical2/1
  Logical2/1 -> new_acc/1

== system satcorr_108/calc_adc_sum_sq ==
  In1 : Inport  Port=1  LatchInput=off
  In2 : Inport  Port=2  LatchInput=off
  In3 : Inport  Port=3  LatchInput=off
  In4 : Inport  Port=4  LatchInput=off
  Accumulator : xbsIndex_r3/Accumulator  n_bits=32  overflow=Wrap  operation=Add  scale=1  explicit_period=off  period=1  rst=on  hasbypass=off  en=off  dbl_ovrd=off  show_param=off  gen_core=off  use_rpm=on
      settings: xl_area=[0, 0, 0, 0, 0, 0, 0]
  Counter : xbsIndex_r3/Counter  cnt_type=Free Running  n_bits=2  bin_pt=0  arith_type=Unsigned  start_count=0  cnt_to=Inf  cnt_by_val=1  operation=Up  explicit_period=off  period=1  load_pin=off  rst=off  en=off  dbl_ovrd=off  show_param=off  use_rpm=on  gen_core=off
      settings: xl_area=[0, 0, 0, 0, 0, 0, 0]
  Counter1 : xbsIndex_r3/Counter  cnt_type=Free Running  n_bits=16  bin_pt=0  arith_type=Unsigned  start_count=0  cnt_to=Inf  cnt_by_val=1  operation=Up  explicit_period=off  period=1  load_pin=off  rst=off  en=off  dbl_ovrd=off  show_param=off  use_rpm=on  gen_core=off
      settings: xl_area=[0, 0, 0, 0, 0, 0, 0]
  Mult : xbsIndex_r3/Mult  precision=Full  arith_type="Signed  (2's comp)"  n_bits=8  bin_pt=2  quantization=Truncate  overflow=Wrap  latency=2  explicit_period=on  period=1  en=off  dbl_ovrd=off  show_param=off  mult_type=Parallel  oversample=2  use_embedded=off  pipeline=on  use_rpm=on  placement_style=Rectangular Shape  gen_core=off
      settings: xl_area=[0, 0, 0, 0, 0, 0, 0]
  Mux : xbsIndex_r3/Mux  inputs=4  precision=Full  arith_type="Signed  (2's comp)"  n_bits=8  bin_pt=2  quantization=Truncate  overflow=Wrap  latency=1  explicit_period=off  period=1  en=off  dbl_ovrd=off  show_param=off  mux_type=off  use_rpm=off  gen_core=off
      settings: xl_area=[0, 0, 0, 0, 0, 0, 0]
  Register : xbsIndex_r3/Register  init=0  reg_only_valid=off  explicit_period=off  period=1  rst=off  en=on  out_en=off  dbl_ovrd=off  show_param=off
      settings: xl_area=[0, 0, 0, 0, 0, 0, 0]
  Slice : xbsIndex_r3/Slice  mode=Upper Bit Location + Width  nbits=1  bit1=0  base1=MSB of Input  bit0=0  base0=LSB of Input  boolean_output=off  explicit_period=off  period=1  dbl_ovrd=off
  negedge : Subsystem
  sum_sq : Outport
  wires:
  Mult/1 -> Accumulator/1
  Accumulator/1 -> Register/1
  Register/1 -> sum_sq/1
  Mux/1 -> Mult/1, Mult/2
  Counter/1 -> Mux/1
  Counter1/1 -> Slice/1
  Slice/1 -> negedge/1(In)
  negedge/1(Out1) -> Accumulator/2, Register/2
  In1/1 -> Mux/2
  In3/1 -> Mux/3
  In2/1 -> Mux/4
  In4/1 -> Mux/5

== system satcorr_108/concat ==
  In1 : Inport  Port=1  LatchInput=off
  In2 : Inport  Port=2  LatchInput=off
  In3 : Inport  Port=3  LatchInput=off
  In4 : Inport  Port=4  LatchInput=off
  Concat2 : xbsIndex_r3/Concat  num_inputs=4  explicit_period=off  period=1  dbl_ovrd=off
  R1 : xbsIndex_r3/Reinterpret  force_arith_type=on  arith_type=Unsigned  force_bin_pt=on  bin_pt=0  force_valid=on
  R2 : xbsIndex_r3/Reinterpret  force_arith_type=on  arith_type=Unsigned  force_bin_pt=on  bin_pt=0  force_valid=on
  R3 : xbsIndex_r3/Reinterpret  force_arith_type=on  arith_type=Unsigned  force_bin_pt=on  bin_pt=0  force_valid=on
  Reinterpret2 : xbsIndex_r3/Reinterpret  force_arith_type=on  arith_type=Unsigned  force_bin_pt=on  bin_pt=0  force_valid=on
  Out1 : Outport
  wires:
  Reinterpret2/1 -> Concat2/1
  R1/1 -> Concat2/2
  R2/1 -> Concat2/3
  R3/1 -> Concat2/4
  In1/1 -> Reinterpret2/1
  In2/1 -> R1/1
  In3/1 -> R2/1
  In4/1 -> R3/1
  Concat2/1 -> Out1/1

== system satcorr_108/concat4 ==
  In1 : Inport  Port=1  LatchInput=off
  In2 : Inport  Port=2  LatchInput=off
  In3 : Inport  Port=3  LatchInput=off
  In4 : Inport  Port=4  LatchInput=off
  Concat2 : xbsIndex_r3/Concat  num_inputs=4  explicit_period=off  period=1  dbl_ovrd=off
  R1 : xbsIndex_r3/Reinterpret  force_arith_type=on  arith_type=Unsigned  force_bin_pt=on  bin_pt=0  force_valid=on
  R2 : xbsIndex_r3/Reinterpret  force_arith_type=on  arith_type=Unsigned  force_bin_pt=on  bin_pt=0  force_valid=on
  R3 : xbsIndex_r3/Reinterpret  force_arith_type=on  arith_type=Unsigned  force_bin_pt=on  bin_pt=0  force_valid=on
  Reinterpret2 : xbsIndex_r3/Reinterpret  force_arith_type=on  arith_type=Unsigned  force_bin_pt=on  bin_pt=0  force_valid=on
  Out1 : Outport
  wires:
  Concat2/1 -> Out1/1
  In4/1 -> R3/1
  In3/1 -> R2/1
  In2/1 -> R1/1
  In1/1 -> Reinterpret2/1
  R3/1 -> Concat2/4
  R2/1 -> Concat2/3
  R1/1 -> Concat2/2
  Reinterpret2/1 -> Concat2/1

== system satcorr_108/concat5 ==
  In1 : Inport  Port=1  LatchInput=off
  In2 : Inport  Port=2  LatchInput=off
  In3 : Inport  Port=3  LatchInput=off
  In4 : Inport  Port=4  LatchInput=off
  Concat2 : xbsIndex_r3/Concat  num_inputs=4  explicit_period=off  period=1  dbl_ovrd=off
  R1 : xbsIndex_r3/Reinterpret  force_arith_type=on  arith_type=Unsigned  force_bin_pt=on  bin_pt=0  force_valid=on
  R2 : xbsIndex_r3/Reinterpret  force_arith_type=on  arith_type=Unsigned  force_bin_pt=on  bin_pt=0  force_valid=on
  R3 : xbsIndex_r3/Reinterpret  force_arith_type=on  arith_type=Unsigned  force_bin_pt=on  bin_pt=0  force_valid=on
  Reinterpret2 : xbsIndex_r3/Reinterpret  force_arith_type=on  arith_type=Unsigned  force_bin_pt=on  bin_pt=0  force_valid=on
  Out1 : Outport
  wires:
  Reinterpret2/1 -> Concat2/1
  R1/1 -> Concat2/2
  R2/1 -> Concat2/3
  R3/1 -> Concat2/4
  In1/1 -> Reinterpret2/1
  In2/1 -> R1/1
  In3/1 -> R2/1
  In4/1 -> R3/1
  Concat2/1 -> Out1/1

== system satcorr_108/concat6 ==
  In1 : Inport  Port=1  LatchInput=off
  In2 : Inport  Port=2  LatchInput=off
  In3 : Inport  Port=3  LatchInput=off
  In4 : Inport  Port=4  LatchInput=off
  Concat2 : xbsIndex_r3/Concat  num_inputs=4  explicit_period=off  period=1  dbl_ovrd=off
  R1 : xbsIndex_r3/Reinterpret  force_arith_type=on  arith_type=Unsigned  force_bin_pt=on  bin_pt=0  force_valid=on
  R2 : xbsIndex_r3/Reinterpret  force_arith_type=on  arith_type=Unsigned  force_bin_pt=on  bin_pt=0  force_valid=on
  R3 : xbsIndex_r3/Reinterpret  force_arith_type=on  arith_type=Unsigned  force_bin_pt=on  bin_pt=0  force_valid=on
  Reinterpret2 : xbsIndex_r3/Reinterpret  force_arith_type=on  arith_type=Unsigned  force_bin_pt=on  bin_pt=0  force_valid=on
  Out1 : Outport
  wires:
  Concat2/1 -> Out1/1
  In4/1 -> R3/1
  In3/1 -> R2/1
  In2/1 -> R1/1
  In1/1 -> Reinterpret2/1
  R3/1 -> Concat2/4
  R2/1 -> Concat2/3
  R1/1 -> Concat2/2
  Reinterpret2/1 -> Concat2/1

== system satcorr_108/decat ==
  In1 : Inport  Port=1  LatchInput=off
  Reinterpret{1..4} (4 alike) : xbsIndex_r3/Reinterpret  force_arith_type=on  arith_type="Signed  (2's comp)"  force_bin_pt=on  bin_pt=7  force_valid=on
  Slice15 : xbsIndex_r3/Slice  mode=Lower Bit Location + Width  nbits=8  bit1=0  base1=MSB of Input  bit0=8  base0=LSB of Input  boolean_output=off  explicit_period=off  period=1  dbl_ovrd=off
  Slice16 : xbsIndex_r3/Slice  mode=Lower Bit Location + Width  nbits=8  bit1=0  base1=MSB of Input  bit0=16  base0=LSB of Input  boolean_output=off  explicit_period=off  period=1  dbl_ovrd=off
  Slice17 : xbsIndex_r3/Slice  mode=Lower Bit Location + Width  nbits=8  bit1=0  base1=MSB of Input  bit0=24  base0=LSB of Input  boolean_output=off  explicit_period=off  period=1  dbl_ovrd=off
  Slice9 : xbsIndex_r3/Slice  mode=Lower Bit Location + Width  nbits=8  bit1=0  base1=MSB of Input  bit0=0  base0=LSB of Input  boolean_output=off  explicit_period=off  period=1  dbl_ovrd=off
  Out1 : Outport
  Out2 : Outport  Port=2
  Out3 : Outport  Port=3
  Out4 : Outport  Port=4
  wires:
  In1/1 -> Slice17/1, Slice16/1, Slice9/1, Slice15/1
  Slice17/1 -> Reinterpret2/1
  Slice16/1 -> Reinterpret1/1
  Slice15/1 -> Reinterpret3/1
  Slice9/1 -> Reinterpret4/1
  Reinterpret2/1 -> Out1/1
  Reinterpret1/1 -> Out2/1
  Reinterpret3/1 -> Out3/1
  Reinterpret4/1 -> Out4/1
